simulink model "UT_simple_gain"  (R2022a)
settings: Solver=VariableStepAuto  StartTime=0.0  StopTime=10.0  RelTol=1e-3
settings Model: Creator=a.dehghan  LastModifiedBy=a.dehghan

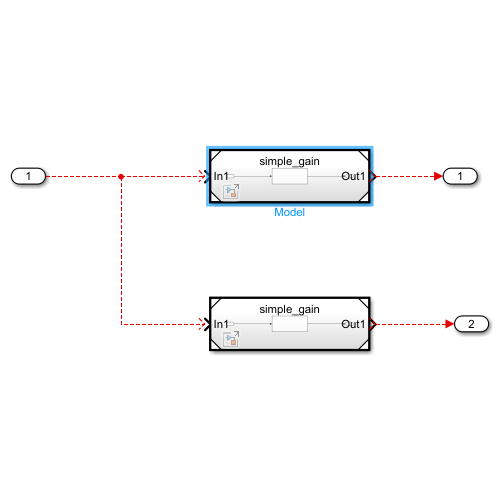
[thumbnail: Simulink's stored preview of the top-level diagram]
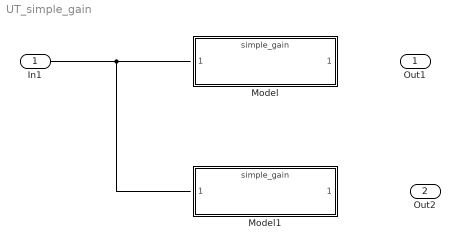
== system UT_simple_gain ==
  In1 : Inport
  Model : ModelReference  ModelNameDialog=simple_gain.slx  UsingDefaultArgumentValue=0  SimulationMode=Normal  ModelReferenceVersion=1.3
  Model1 : ModelReference  ModelNameDialog=simple_gain.slx  UsingDefaultArgumentValue=0  SimulationMode=Normal  ModelReferenceVersion=1.3
  Out1 : Outport
  Out2 : Outport  Port=2
  wires:
  In1/1 -> ?
  ? -> Out1/1
  ? -> Out2/1
